simulink subsystem "selector"  (R2023a)
settings: Solver=VariableStepAuto  StartTime=0.0  StopTime=10.0  RelTol=1e-3
settings Model: Creator=mergurtu  LastModifiedBy=mergurtu

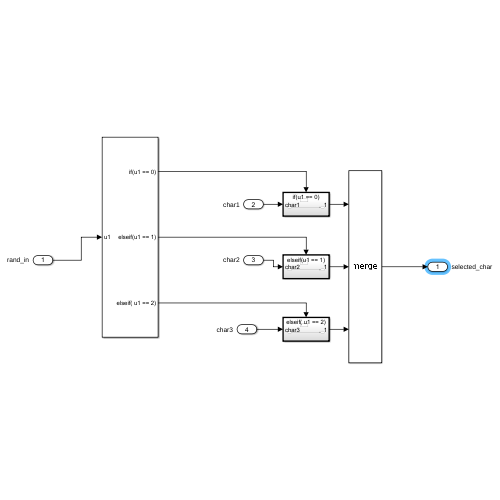
[thumbnail: Simulink's stored preview of the top-level diagram]
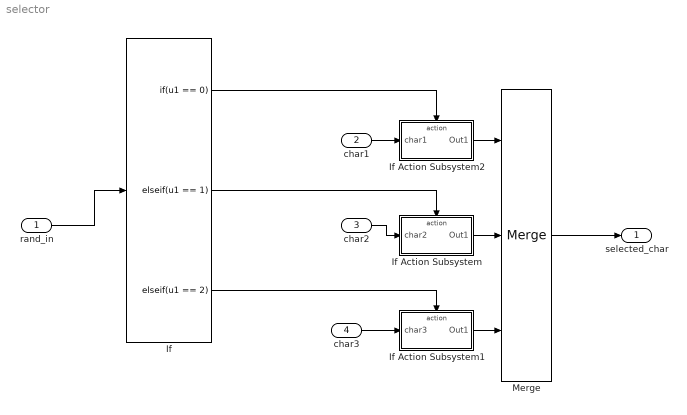
== system selector ==
  rand_in : Inport  OutDataTypeStr=uint8
  char1 : Inport  Port=2  OutDataTypeStr=uint8
  char2 : Inport  Port=3  OutDataTypeStr=uint8
  char3 : Inport  Port=4  OutDataTypeStr=uint8
  If : If  IfExpression=u1 == 0  ElseIfExpressions=u1 == 1, u1 == 2  ShowElse=off
  If Action Subsystem : Subsystem  TreatAsAtomicUnit=on
  If Action Subsystem1 : Subsystem  TreatAsAtomicUnit=on
  If Action Subsystem2 : Subsystem  TreatAsAtomicUnit=on
  Merge : Merge  Inputs=3
  selected_char : Outport  OutDataTypeStr=uint8
  wires:
  char1/1 -> If Action Subsystem2/1(char1)
  char2/1 -> If Action Subsystem/1(char2)
  rand_in/1 -> If/1
  char3/1 -> If Action Subsystem1/1(char3)
  Merge/1 -> selected_char/1
  If/1 -> If Action Subsystem2/Action
  If/2 -> If Action Subsystem/Action
  If/3 -> If Action Subsystem1/Action
  If Action Subsystem2/1(Out1) -> Merge/1
  If Action Subsystem/1(Out1) -> Merge/2
  If Action Subsystem1/1(Out1) -> Merge/3

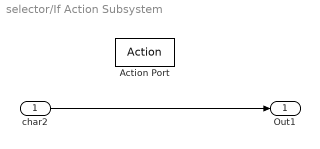
== system selector/If Action Subsystem ==
  char2 : Inport
  Action Port : ActionPort  ActionPortLabel=elseif(u1 == 1)
  Out1 : Outport
  wires:
  char2/1 -> Out1/1

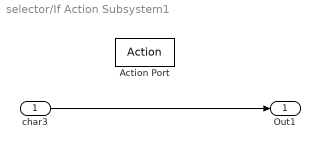
== system selector/If Action Subsystem1 ==
  char3 : Inport
  Action Port : ActionPort  ActionPortLabel=elseif( u1 == 2)
  Out1 : Outport
  wires:
  char3/1 -> Out1/1

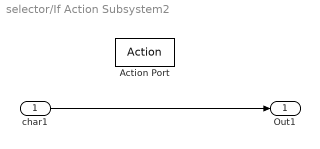
== system selector/If Action Subsystem2 ==
  char1 : Inport
  Action Port : ActionPort  ActionPortLabel=if(u1 == 0)
  Out1 : Outport
  wires:
  char1/1 -> Out1/1
